simulink library "BLDC_controller_Lib_AccelerationBased"  (R2017b)
settings: Solver=VariableStepAuto  StartTime=0.0  StopTime=10.0  RelTol=1e-3
values from neighbouring files (symbols this model uses):
  a_elecAngle = 60    [init_model_Ffwd.m]
  a_elecPeriod = 360    [init_model_Ffwd.m]
  cf_speedCoef = round(f_ctrl * a_mechAngle * (pi/180) * (30/pi))    [init_model_Ffwd.m]
  cf_speedFilt = 0.20    (= 0.2)    [init_model_Ffwd.m]
  n_commAcvLo = 15    [init_model_Ffwd.m]
  n_commDeacvHi = 30    [init_model_Ffwd.m]
  r_sinPhaA_M1 = -sca_factor*sin(omega + pha_adv*(pi/180))    [init_model_Ffwd.m]
  r_sinPhaB_M1 = -sca_factor*sin(omega - 120*(pi/180) + pha_adv*(pi/180))    [init_model_Ffwd.m]
  r_sinPhaC_M1 = -sca_factor*sin(omega + 120*(pi/180) + pha_adv*(pi/180))    [init_model_Ffwd.m]
  r_trapPhaA_M1 = sca_factor*[ 1  1  1 -1 -1 -1  1]    [init_model_Ffwd.m]
  r_trapPhaB_M1 = sca_factor*[-1 -1  1  1  1 -1 -1]    [init_model_Ffwd.m]
  r_trapPhaC_M1 = sca_factor*[ 1 -1 -1 -1  1  1  1]    [init_model_Ffwd.m]
  vec_hallToPos = [0 2 0 1 4 3 5 0]    [init_model_Ffwd.m]
  z_commutMap_M1 = [-1 -1  0  1  1  0 ... (first row only)    [init_model_Ffwd.m]
  z_ctrlTypSel = 1    [init_model_Ffwd.m]
  z_maxCntRst = 2000    [init_model_Ffwd.m]
undefined symbols (not defined in the file or in its folder): a_phaAdv_M1, b_phaAdvEna, cf_speedSca, CTRL_COMM, r_commDCDeacv, r_sin3PhaA_M1, r_sin3PhaB_M1, r_sin3PhaC_M1, z_nrEdgeSpdAcv
libraries: BLDC_controller_Lib x3, simulink_extras x1
settings Model: Creator=37ef  LastModifiedBy=37ef

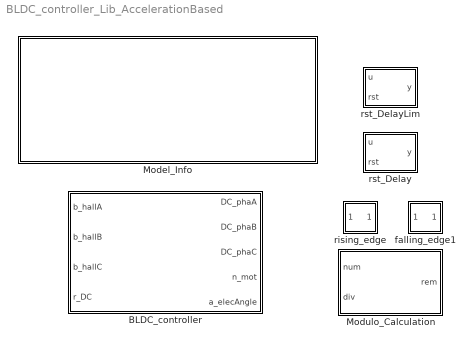
== system BLDC_controller_Lib_AccelerationBased ==
  BLDC_controller : Subsystem  SystemSampleTime=1e-5
  Model_Info : Subsystem
      mask DialogControl DescGroupVar Prompt: Model info
      mask DialogControl DescTextVar Prompt: This mask gives quick information about the model.
      mask Display:
      | info = Simulink.MDLInfo(bdroot);
      | file = dir([bdroot '.slx']);
      | % image('logo.png', [0.48, 0.55, 0.5, 0.4]);
      | text(0.05, 0.5, [...
      |         'MODEL INFO \n\n' ...
      |         'Version: ' info.ModelVersion '\n' ...
      |         'Author: ' 'Emanuel Feru' '\n' ...
      |         'Last modified by: ' info.LastModifiedBy '\n' ...
      |         'Last update: ' file.date '\n\n'], ...
      |         'horizontalAlignment', 'left', ...
      |         'verticalAlignment', 'middle');
      | 
      | color('blue');
      | text(0.95, 0.08, [...
      |         'Copyright © 2019 Emanuel FERU'], ...
      |         'horizontalAlignment', 'right', ...
      |         'verticalAlignment', 'bottom');
  Modulo_Calculation : Subsystem
  falling_edge1 : Subsystem  StopFcn=%tagged  TreatAsAtomicUnit=on  mask(Falling edge detection){}
      mask help:
      | Falling edge detection for a logic signal.
      | When a falling edge on the input signal is detected, the output switches to 1 during one time step.
      settings: RTWSystemCode=Nonreusable function
      mask Display: plot(0,0,100,100, [20 50 50 80], [90 90 10 10], [40 50 60], [55 45 55] )
  rising_edge : Subsystem  StopFcn=%tagged  TreatAsAtomicUnit=on  mask(Rising edge detection){}
      mask help:
      | Rising edge detection for a logic signal.
      | When a rising edge on the input signal is detected, the output switches to 1 during one time step.
      settings: RTWSystemCode=Nonreusable function
      mask Display: plot(0,0,100,100, [20 50 50 80], [10 10 90 90], [40 50 60], [45 55 45] )
  rst_Delay : Subsystem
      mask Display: dpoly(1,[1 0],'z')
  rst_DelayLim : Subsystem  mask{z_cntMaxLim=200}
      mask prompts: z_cntMaxLim "Maximum counter limit"
      mask Display: dpoly(1,[1 0],'z')

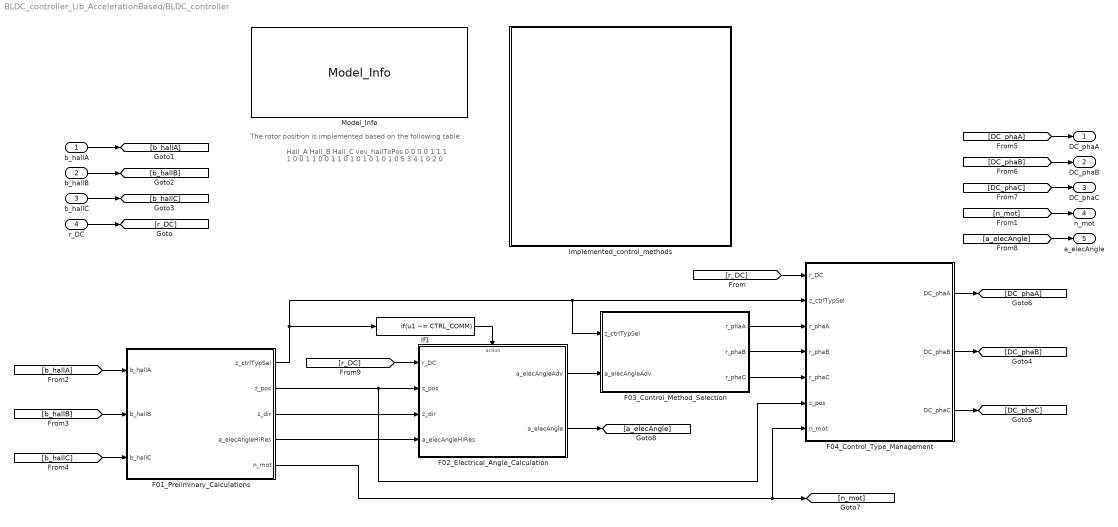
== system BLDC_controller_Lib_AccelerationBased/BLDC_controller ==
  note: The rotor position is implemented based on the following table:
  note: Hall_A
      | Hall_B
      | Hall_C
      | vev_hallToPos
      |
      | 0
      | 0
      | 0
      | 0
      | 1
      | 1
      | 1
      | 1
      | 0
      | 0
      | 1
      | 1
      | 0
      | 0
      | 1
      | 1
      | 0
      | 1
      | 0
      | 1
      | 0
      | 1
      | 0
      | 1
      | 0
      | 5
      | 3
      | 4
      | 1
      | 0
      | 2
      | 0
  "b_hallA " : Inport
  b_hallB : Inport  Port=2
  b_hallC : Inport  Port=3
  r_DC : Inport  Port=4
  F01_Preliminary_Calculations : Subsystem
  F02_Electrical_Angle_Calculation : Subsystem
  F03_Control_Method_Selection : Subsystem
  F04_Control_Type_Management : Subsystem
  If1 : If  IfExpression=u1 ~= CTRL_COMM  ShowElse=off
  Implemented_control_methods : Subsystem
      mask Display: image('control_methods.png')
  Model_Info : BLDC_controller_Lib/Model_Info
  DC_phaA : Outport
  DC_phaB : Outport  Port=2
  DC_phaC : Outport  Port=3
  n_mot : Outport  Port=4
  a_elecAngle : Outport  Port=5
  wires:
  "b_hallA "/1 -> [b_hallA]
  b_hallB/1 -> [b_hallB]
  b_hallC/1 -> [b_hallC]
  [n_mot] -> n_mot/1
  [DC_phaA] -> DC_phaA/1
  [b_hallA] -> F01_Preliminary_Calculations/1(b_hallA)
  [b_hallC] -> F01_Preliminary_Calculations/3(b_hallC)
  [b_hallB] -> F01_Preliminary_Calculations/2(b_hallB)
  F01_Preliminary_Calculations/2(z_pos) -> F04_Control_Type_Management/6(z_pos), F02_Electrical_Angle_Calculation/2(z_pos)
  F01_Preliminary_Calculations/3(z_dir) -> F02_Electrical_Angle_Calculation/3(z_dir)
  F01_Preliminary_Calculations/5("n_mot ") -> F04_Control_Type_Management/7(n_mot), [n_mot]
  F01_Preliminary_Calculations/4(a_elecAngleHiRes) -> F02_Electrical_Angle_Calculation/4(a_elecAngleHiRes)
  F01_Preliminary_Calculations/1(z_ctrlTypSel) -> F04_Control_Type_Management/2(z_ctrlTypSel), F03_Control_Method_Selection/1(z_ctrlTypSel), If1/1
  If1/1 -> F02_Electrical_Angle_Calculation/Action
  F02_Electrical_Angle_Calculation/1(a_elecAngleAdv) -> F03_Control_Method_Selection/2(a_elecAngleAdv)
  F03_Control_Method_Selection/1(r_phaA) -> F04_Control_Type_Management/3(r_phaA)
  F03_Control_Method_Selection/2(r_phaB) -> F04_Control_Type_Management/4(r_phaB)
  F03_Control_Method_Selection/3("r_phaC ") -> F04_Control_Type_Management/5(r_phaC)
  [r_DC] -> F04_Control_Type_Management/1(r_DC)
  F04_Control_Type_Management/1(DC_phaA) -> [DC_phaA]
  F04_Control_Type_Management/2(DC_phaB) -> [DC_phaB]
  F04_Control_Type_Management/3("DC_phaC ") -> [DC_phaC]
  [DC_phaB] -> DC_phaB/1
  [DC_phaC] -> DC_phaC/1
  r_DC/1 -> [r_DC]
  [a_elecAngle] -> a_elecAngle/1
  F02_Electrical_Angle_Calculation/2(a_elecAngle) -> [a_elecAngle]
  [r_DC] -> F02_Electrical_Angle_Calculation/1(r_DC)

== system BLDC_controller_Lib_AccelerationBased/Model_Info ==

== system BLDC_controller_Lib_AccelerationBased/Modulo_Calculation ==
  note: Modulo implementation: rem = num - div*(num/div)
      | Note : Division and multiplier has the setting 'Floor'
  num : Inport
  div : Inport  Port=2
  Divide2 : Product  Inputs=*/  OutDataTypeStr=Inherit: Same as first input
  Divide3 : Product  Inputs=**  OutDataTypeStr=Inherit: Same as first input
  Sum3 : Sum  Inputs=|+-  RndMeth=Simplest  OutDataTypeStr=Inherit: Same as first input
  rem : Outport
  wires:
  num/1 -> Sum3/1, Divide2/1
  Sum3/1 -> rem/1
  Divide3/1 -> Sum3/2
  div/1 -> Divide3/2, Divide2/2
  Divide2/1 -> Divide3/1

== system BLDC_controller_Lib_AccelerationBased/falling_edge1 ==
  Signal : Inport
  Logical Operator : Logic  Tag=struct('inputs','2','comment',struct('text','','placement',1),'logdata',struct('maxnumvals',inf,'plotchannels',[],'loggingmode',3,'channels',1),'operator','AND','output',struct('variable','','description','','name','$S_$B','address','','class','default','type','Bool','unit',''),'scalingvalid',0,'date',733067.68453166669)  OutDataTypeStr=boolean
  Logical Operator1 : Logic  Tag=struct('inputs','1','comment',struct('text','','placement',1),'logdata',struct('maxnumvals',inf,'plotchannels',[],'loggingmode',3,'channels',1),'operator','NOT','output',struct('variable','','description','','name','$S_$B','address','','class','default','type','Bool','unit',''),'scalingvalid',0,'date',733067.68453201384)  Operator=NOT  Inputs=1  OutDataTypeStr=boolean
  UnitDelay : UnitDelay  SampleTime=-1
      settings: AttributesFormatString=Te = %<SampleTime>\nIni=%<X0>
  Out : Outport
  wires:
  UnitDelay/1 -> Logical Operator/2
  Logical Operator1/1 -> Logical Operator/1
  Signal/1 -> UnitDelay/1, Logical Operator1/1
  Logical Operator/1 -> Out/1

== system BLDC_controller_Lib_AccelerationBased/rising_edge ==
  Signal : Inport
  Logical Operator : Logic  Tag=struct('inputs','2','comment',struct('text','','placement',1),'logdata',struct('maxnumvals',inf,'plotchannels',[],'loggingmode',3,'channels',1),'operator','AND','output',struct('variable','','description','','name','$S_$B','address','','class','default','type','Bool','unit',''),'scalingvalid',0,'date',733067.68458487268)  OutDataTypeStr=boolean
  Logical Operator1 : Logic  Tag=struct('inputs','1','comment',struct('text','','placement',1),'logdata',struct('maxnumvals',inf,'plotchannels',[],'loggingmode',3,'channels',1),'operator','NOT','output',struct('variable','','description','','name','$S_$B','address','','class','default','type','Bool','unit',''),'scalingvalid',0,'date',733067.68458533566)  Operator=NOT  Inputs=1  OutDataTypeStr=boolean
  UnitDelay : UnitDelay  SampleTime=-1
      settings: AttributesFormatString=Te = %<SampleTime>\nIni=%<X0>
  Out : Outport
  wires:
  UnitDelay/1 -> Logical Operator1/1
  Logical Operator1/1 -> Logical Operator/2
  Signal/1 -> Logical Operator/1, UnitDelay/1
  Logical Operator/1 -> Out/1

== system BLDC_controller_Lib_AccelerationBased/rst_Delay ==
  u : Inport
  rst : Inport  Port=2
  Constant23 : Constant  Value=0  OutDataTypeStr=Inherit: Inherit via back propagation
  Switch1 : Switch  Criteria=u2 ~= 0  OutDataTypeStr=Inherit: Inherit via back propagation  RndMeth=Simplest
  UnitDelay1 : UnitDelay  SampleTime=-1
  y : Outport
  wires:
  Switch1/1 -> y/1
  u/1 -> UnitDelay1/1
  UnitDelay1/1 -> Switch1/3
  rst/1 -> Switch1/2
  Constant23/1 -> Switch1/1

== system BLDC_controller_Lib_AccelerationBased/rst_DelayLim ==
  u : Inport
  rst : Inport  Port=2
  Constant1 : Constant  Value=z_cntMaxLim  OutDataTypeStr=Inherit: Inherit via back propagation
  Constant23 : Constant  Value=0  OutDataTypeStr=Inherit: Inherit via back propagation
  Relational Operator1 : RelationalOperator  Operator=<  OutDataTypeStr=boolean  RndMeth=Simplest
  Switch1 : Switch  Criteria=u2 ~= 0  OutDataTypeStr=Inherit: Inherit via back propagation  RndMeth=Simplest
  Switch2 : Switch  Criteria=u2 ~= 0  OutDataTypeStr=Inherit: Inherit via back propagation  RndMeth=Simplest
  UnitDelay1 : UnitDelay  InitialCondition=z_cntMaxLim  SampleTime=-1
  y : Outport
  wires:
  Switch1/1 -> y/1
  u/1 -> UnitDelay1/1
  rst/1 -> Switch1/2
  Constant23/1 -> Switch1/1
  UnitDelay1/1 -> Switch2/1, Relational Operator1/1
  Constant1/1 -> Switch2/3, Relational Operator1/2
  Relational Operator1/1 -> Switch2/2
  Switch2/1 -> Switch1/3

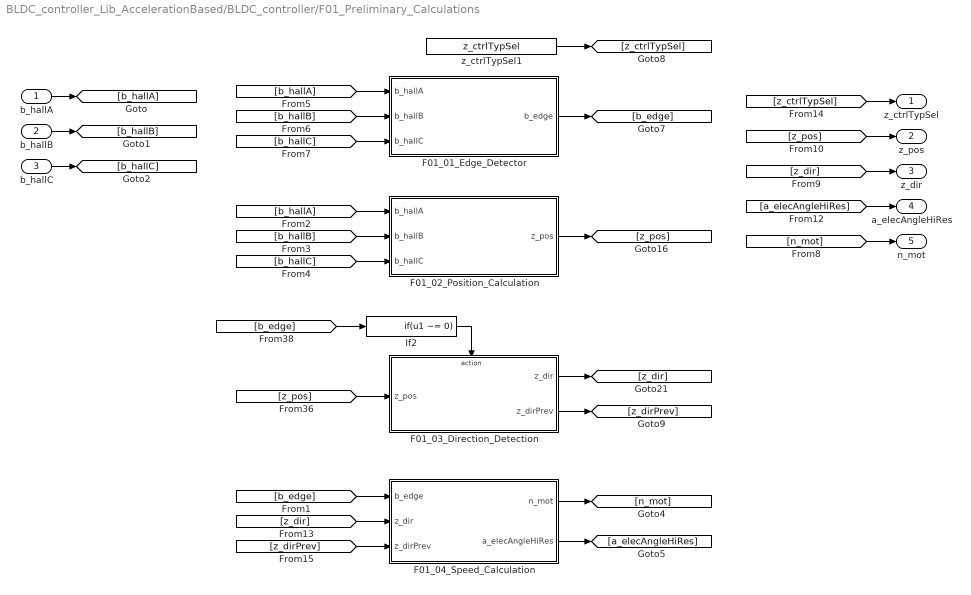
== system BLDC_controller_Lib_AccelerationBased/BLDC_controller/F01_Preliminary_Calculations ==
  b_hallA : Inport
  b_hallB : Inport  Port=2
  b_hallC : Inport  Port=3
  F01_01_Edge_Detector : Subsystem
  F01_02_Position_Calculation : Subsystem
  F01_03_Direction_Detection : Subsystem
  F01_04_Speed_Calculation : Subsystem
  If2 : If  IfExpression=u1 ~= 0  ShowElse=off
  z_ctrlTypSel1 : Constant  Value=z_ctrlTypSel  OutDataTypeStr=uint8
  z_ctrlTypSel : Outport  OutputWhenDisabled=reset  InitialOutput=0
  z_pos : Outport  Port=2  OutputWhenDisabled=reset  InitialOutput=0
  z_dir : Outport  Port=3  OutputWhenDisabled=reset  InitialOutput=0
  a_elecAngleHiRes : Outport  Port=4  OutputWhenDisabled=reset  InitialOutput=0
  "n_mot " : Outport  Port=5  OutputWhenDisabled=reset  InitialOutput=0
  wires:
  If2/1 -> F01_03_Direction_Detection/Action
  [b_edge] -> If2/1
  [z_pos] -> F01_03_Direction_Detection/1(z_pos)
  [b_hallA] -> F01_01_Edge_Detector/1(b_hallA)
  F01_01_Edge_Detector/1("b_edge ") -> [b_edge]
  F01_03_Direction_Detection/1(z_dir) -> [z_dir]
  [b_hallB] -> F01_01_Edge_Detector/2(b_hallB)
  [b_hallC] -> F01_01_Edge_Detector/3(b_hallC)
  b_hallA/1 -> [b_hallA]
  b_hallB/1 -> [b_hallB]
  b_hallC/1 -> [b_hallC]
  [b_hallC] -> F01_02_Position_Calculation/3(b_hallC)
  [b_hallB] -> F01_02_Position_Calculation/2(b_hallB)
  [b_hallA] -> F01_02_Position_Calculation/1(b_hallA)
  F01_02_Position_Calculation/1("z_pos ") -> [z_pos]
  [b_edge] -> F01_04_Speed_Calculation/1(b_edge)
  F01_04_Speed_Calculation/1(n_mot) -> [n_mot]
  [n_mot] -> "n_mot "/1
  [z_dir] -> z_dir/1
  [z_pos] -> z_pos/1
  F01_04_Speed_Calculation/2(a_elecAngleHiRes) -> [a_elecAngleHiRes]
  [a_elecAngleHiRes] -> a_elecAngleHiRes/1
  [z_dir] -> F01_04_Speed_Calculation/2(z_dir)
  [z_ctrlTypSel] -> z_ctrlTypSel/1
  z_ctrlTypSel1/1 -> [z_ctrlTypSel]
  F01_03_Direction_Detection/2(z_dirPrev) -> [z_dirPrev]
  [z_dirPrev] -> F01_04_Speed_Calculation/3(z_dirPrev)

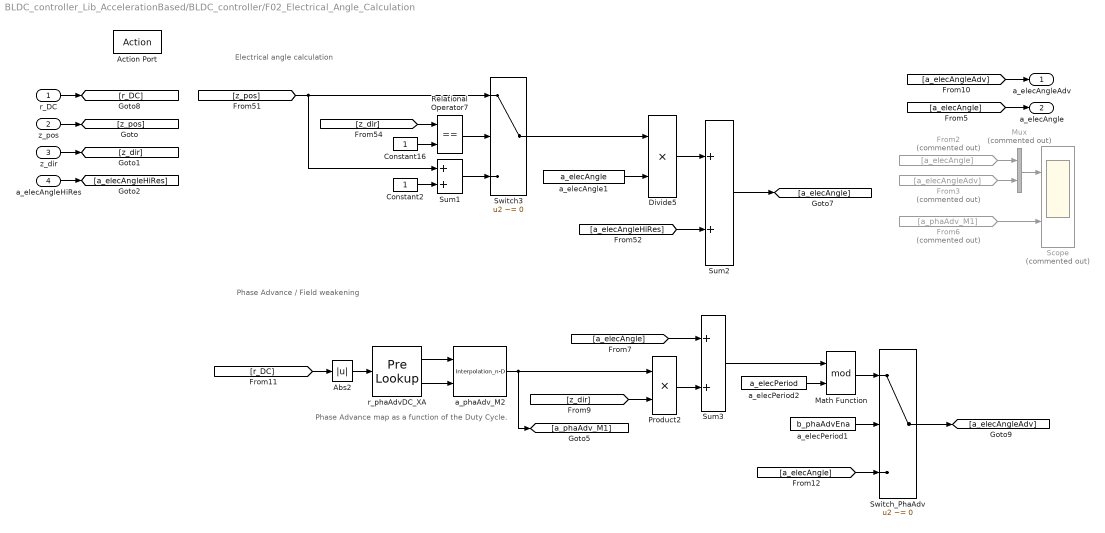
== system BLDC_controller_Lib_AccelerationBased/BLDC_controller/F02_Electrical_Angle_Calculation ==
  note: Electrical angle calculation
  note: Phase Advance / Field weakening
  note: Phase Advance map as a function of the Duty Cycle.
  r_DC : Inport
  z_pos : Inport  Port=2
  z_dir : Inport  Port=3
  a_elecAngleHiRes : Inport  Port=4
  Action Port : ActionPort
  Abs2 : Abs  ZeroCross=off  OutDataTypeStr=Inherit: Inherit via back propagation  RndMeth=Simplest
  Constant16 : Constant  OutDataTypeStr=Inherit: Inherit via back propagation
  Constant2 : Constant  OutDataTypeStr=Inherit: Inherit via back propagation
  Divide5 : Product  Inputs=**  OutDataTypeStr=int32  RndMeth=Simplest
  From2 : From  Commented=on  GotoTag=a_elecAngle
  From3 : From  Commented=on  GotoTag=a_elecAngleAdv
  From6 : From  Commented=on  GotoTag=a_phaAdv_M1
  Math Function : Math  Operator=mod  SaturateOnIntegerOverflow=on
  Mux : Mux  Commented=on  Inputs=2
  Product2 : Product  RndMeth=Simplest  OutDataTypeStr=Inherit: Same as first input
  Relational Operator7 : RelationalOperator  Operator===  OutDataTypeStr=boolean  RndMeth=Simplest
  Scope : Scope  Commented=on  NumInputPorts=2
  Sum1 : Sum  RndMeth=Simplest  OutDataTypeStr=Inherit: Same as first input
  Sum2 : Sum  RndMeth=Simplest  OutDataTypeStr=Inherit: Same as first input
  Sum3 : Sum  RndMeth=Simplest  OutDataTypeStr=Inherit: Same as first input
  Switch3 : Switch  Criteria=u2 ~= 0  OutDataTypeStr=Inherit: Inherit via back propagation  RndMeth=Zero
  Switch_PhaAdv : Switch  Criteria=u2 ~= 0  OutDataTypeStr=Inherit: Inherit via back propagation  RndMeth=Zero
  a_elecAngle1 : Constant  Value=a_elecAngle  OutDataTypeStr=int32
  a_elecPeriod1 : Constant  Value=b_phaAdvEna  OutDataTypeStr=boolean
  a_elecPeriod2 : Constant  Value=a_elecPeriod  OutDataTypeStr=Inherit: Inherit via back propagation
  a_phaAdv_M2 : Interpolation_n-D  NumberOfTableDimensions=1  Table=a_phaAdv_M1  ExtrapMethod=Clip  OutDataTypeStr=int16  InternalRulePriority=Speed  RndMeth=Simplest
      settings: InputPortMap=u0,u1
  r_phaAdvDC_XA : PreLookup  BreakpointsData=r_phaAdvDC_XA  IndexSearchMethod=Evenly spaced points  BeginIndexSearchUsingPreviousIndexResult=on  IndexDataTypeStr=uint8  RndMeth=Simplest
  a_elecAngleAdv : Outport  OutputWhenDisabled=reset  InitialOutput=0
  a_elecAngle : Outport  Port=2  OutputWhenDisabled=reset  InitialOutput=0
  wires:
  a_phaAdv_M2/1 -> [a_phaAdv_M1], Product2/1
  [z_dir] -> Product2/2
  [a_elecAngleHiRes] -> Sum2/2
  z_pos/1 -> [z_pos]
  z_dir/1 -> [z_dir]
  a_elecAngleHiRes/1 -> [a_elecAngleHiRes]
  Switch3/1 -> Divide5/1
  [z_pos] -> Sum1/1, Switch3/1
  Relational Operator7/1 -> Switch3/2
  [z_dir] -> Relational Operator7/1
  Divide5/1 -> Sum2/1
  Constant16/1 -> Relational Operator7/2
  a_elecAngle1/1 -> Divide5/2
  Constant2/1 -> Sum1/2
  Sum2/1 -> [a_elecAngle]
  Mux/1 -> Scope/1
  From2/1 -> Mux/1
  From3/1 -> Mux/2
  Sum1/1 -> Switch3/3
  [a_elecAngle] -> a_elecAngle/1
  [a_elecAngleAdv] -> a_elecAngleAdv/1
  From6/1 -> Scope/2
  a_elecPeriod1/1 -> Switch_PhaAdv/2
  r_phaAdvDC_XA/2 -> a_phaAdv_M2/2
  r_phaAdvDC_XA/1 -> a_phaAdv_M2/1
  [a_elecAngle] -> Switch_PhaAdv/3
  r_DC/1 -> [r_DC]
  Switch_PhaAdv/1 -> [a_elecAngleAdv]
  Product2/1 -> Sum3/2
  [a_elecAngle] -> Sum3/1
  [r_DC] -> Abs2/1
  Abs2/1 -> r_phaAdvDC_XA/1
  a_elecPeriod2/1 -> Math Function/2
  Math Function/1 -> Switch_PhaAdv/1
  Sum3/1 -> Math Function/1

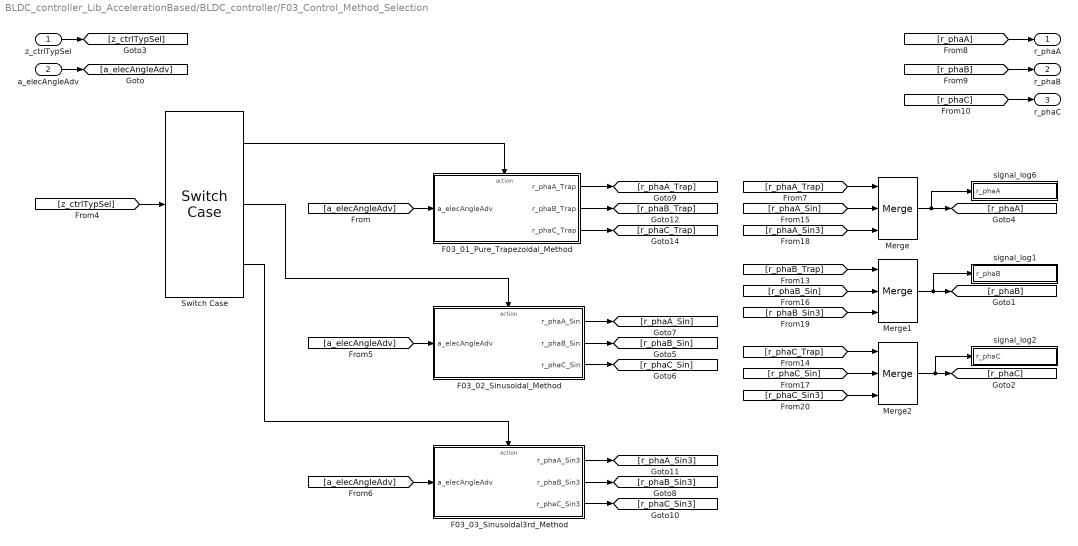
== system BLDC_controller_Lib_AccelerationBased/BLDC_controller/F03_Control_Method_Selection ==
  z_ctrlTypSel : Inport
  a_elecAngleAdv : Inport  Port=2
  F03_01_Pure_Trapezoidal_Method : Subsystem
  F03_02_Sinusoidal_Method : Subsystem
  F03_03_Sinusoidal3rd_Method : Subsystem
  Merge : Merge  Inputs=3
  Merge1 : Merge  Inputs=3
  Merge2 : Merge  Inputs=3
  Switch Case : SwitchCase  CaseConditions={CTRL_TRAP, CTRL_SIN, CTRL_SIN3}  ShowDefaultCase=off
  signal_log1 : Subsystem
  signal_log2 : Subsystem
  signal_log6 : Subsystem
  r_phaA : Outport  OutputWhenDisabled=reset  InitialOutput=0
  r_phaB : Outport  Port=2  OutputWhenDisabled=reset  InitialOutput=0
  "r_phaC " : Outport  Port=3  OutputWhenDisabled=reset  InitialOutput=0
  wires:
  [r_phaA] -> r_phaA/1
  [r_phaB] -> r_phaB/1
  [r_phaC] -> "r_phaC "/1
  a_elecAngleAdv/1 -> [a_elecAngleAdv]
  F03_01_Pure_Trapezoidal_Method/1(r_phaA_Trap) -> [r_phaA_Trap]
  [z_ctrlTypSel] -> Switch Case/1
  [a_elecAngleAdv] -> F03_01_Pure_Trapezoidal_Method/1(a_elecAngleAdv)
  Switch Case/1 -> F03_01_Pure_Trapezoidal_Method/Action
  [a_elecAngleAdv] -> F03_02_Sinusoidal_Method/1(a_elecAngleAdv)
  [a_elecAngleAdv] -> F03_03_Sinusoidal3rd_Method/1(a_elecAngleAdv)
  Switch Case/2 -> F03_02_Sinusoidal_Method/Action
  Switch Case/3 -> F03_03_Sinusoidal3rd_Method/Action
  F03_01_Pure_Trapezoidal_Method/2(r_phaB_Trap) -> [r_phaB_Trap]
  F03_01_Pure_Trapezoidal_Method/3(r_phaC_Trap) -> [r_phaC_Trap]
  F03_02_Sinusoidal_Method/3(r_phaC_Sin) -> [r_phaC_Sin]
  F03_02_Sinusoidal_Method/2(r_phaB_Sin) -> [r_phaB_Sin]
  F03_02_Sinusoidal_Method/1(r_phaA_Sin) -> [r_phaA_Sin]
  F03_03_Sinusoidal3rd_Method/3(r_phaC_Sin3) -> [r_phaC_Sin3]
  F03_03_Sinusoidal3rd_Method/2(r_phaB_Sin3) -> [r_phaB_Sin3]
  F03_03_Sinusoidal3rd_Method/1(r_phaA_Sin3) -> [r_phaA_Sin3]
  Merge/1 -> signal_log6/1(r_phaA), [r_phaA]
  Merge1/1 -> signal_log1/1(r_phaB), [r_phaB]
  Merge2/1 -> signal_log2/1(r_phaC), [r_phaC]
  [r_phaA_Trap] -> Merge/1
  z_ctrlTypSel/1 -> [z_ctrlTypSel]
  [r_phaA_Sin] -> Merge/2
  [r_phaA_Sin3] -> Merge/3
  [r_phaB_Trap] -> Merge1/1
  [r_phaB_Sin] -> Merge1/2
  [r_phaC_Trap] -> Merge2/1
  [r_phaB_Sin3] -> Merge1/3
  [r_phaC_Sin] -> Merge2/2
  [r_phaC_Sin3] -> Merge2/3

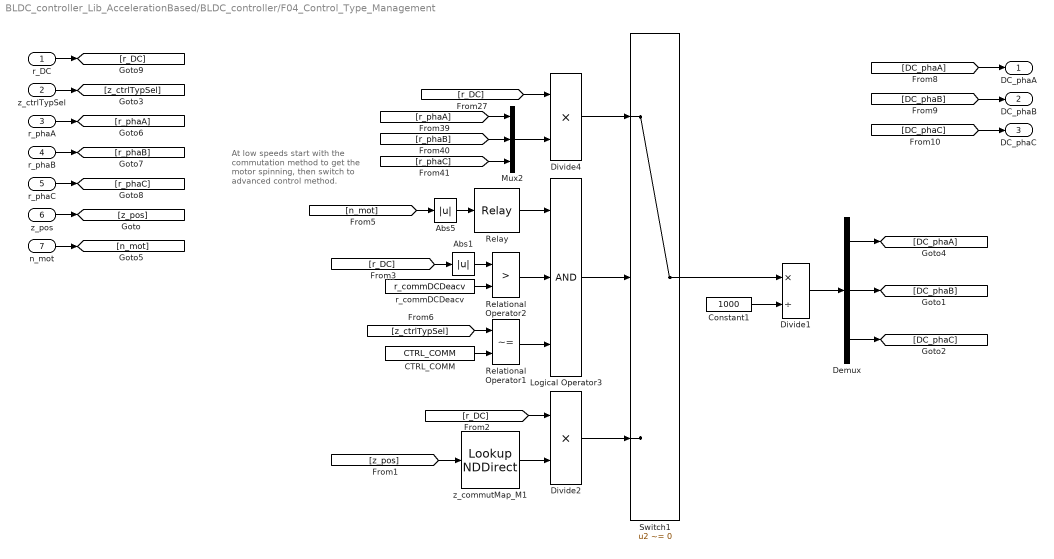
== system BLDC_controller_Lib_AccelerationBased/BLDC_controller/F04_Control_Type_Management ==
  note: At low speeds start with the commutation method to get the motor spinning, then switch to advanced control method.
  r_DC : Inport
  z_ctrlTypSel : Inport  Port=2
  r_phaA : Inport  Port=3
  r_phaB : Inport  Port=4
  r_phaC : Inport  Port=5
  z_pos : Inport  Port=6
  n_mot : Inport  Port=7
  Abs1 : Abs  OutDataTypeStr=Inherit: Inherit via back propagation  RndMeth=Zero
  Abs5 : Abs  OutDataTypeStr=Inherit: Inherit via back propagation  RndMeth=Zero
  CTRL_COMM : Constant  Value=CTRL_COMM  OutDataTypeStr=Inherit: Inherit via back propagation
  Constant1 : Constant  Value=1000  OutDataTypeStr=Inherit: Inherit via back propagation
  Demux : Demux  Outputs=3
  Divide1 : Product  Inputs=*/  RndMeth=Simplest  OutDataTypeStr=Inherit: Same as first input
  Divide2 : Product  Inputs=**  RndMeth=Simplest  OutDataTypeStr=Inherit: Same as first input
  Divide4 : Product  Inputs=**  RndMeth=Simplest  OutDataTypeStr=Inherit: Same as first input
  Logical Operator3 : Logic  Inputs=3  AllPortsSameDT=off  OutDataTypeStr=boolean
  Mux2 : Mux  Inputs=3
  Relational Operator1 : RelationalOperator  Operator=~=  OutDataTypeStr=boolean  RndMeth=Simplest
  Relational Operator2 : RelationalOperator  Operator=>  OutDataTypeStr=boolean  RndMeth=Simplest
  Relay : Relay  OnSwitchValue=n_commDeacvHi  OffSwitchValue=n_commAcvLo  OutDataTypeStr=boolean
  Switch1 : Switch  Criteria=u2 ~= 0  OutDataTypeStr=Inherit: Inherit via back propagation  RndMeth=Zero
  r_commDCDeacv : Constant  Value=r_commDCDeacv  OutDataTypeStr=Inherit: Inherit via back propagation
  z_commutMap_M1 : LookupNDDirect  InputsSelectThisObjectFromTable=Column  Table=z_commutMap_M1  DiagnosticForOutOfRangeInput=None  TableDataTypeStr=int16
  DC_phaA : Outport  OutputWhenDisabled=reset  InitialOutput=0
  DC_phaB : Outport  Port=2  OutputWhenDisabled=reset  InitialOutput=0
  "DC_phaC " : Outport  Port=3  OutputWhenDisabled=reset  InitialOutput=0
  wires:
  z_ctrlTypSel/1 -> [z_ctrlTypSel]
  Demux/3 -> [DC_phaC]
  Demux/2 -> [DC_phaB]
  Demux/1 -> [DC_phaA]
  z_pos/1 -> [z_pos]
  [DC_phaC] -> "DC_phaC "/1
  [DC_phaB] -> DC_phaB/1
  [DC_phaA] -> DC_phaA/1
  Switch1/1 -> Divide1/1
  Relay/1 -> Logical Operator3/1
  [z_ctrlTypSel] -> Relational Operator1/1
  CTRL_COMM/1 -> Relational Operator1/2
  Abs5/1 -> Relay/1
  [z_pos] -> z_commutMap_M1/1
  Divide1/1 -> Demux/1
  n_mot/1 -> [n_mot]
  r_phaA/1 -> [r_phaA]
  r_phaB/1 -> [r_phaB]
  r_phaC/1 -> [r_phaC]
  r_DC/1 -> [r_DC]
  [r_phaA] -> Mux2/1
  [r_phaB] -> Mux2/2
  [r_phaC] -> Mux2/3
  Mux2/1 -> Divide4/2
  Divide4/1 -> Switch1/1
  Constant1/1 -> Divide1/2
  [r_DC] -> Divide2/1
  z_commutMap_M1/1 -> Divide2/2
  Divide2/1 -> Switch1/3
  [n_mot] -> Abs5/1
  Logical Operator3/1 -> Switch1/2
  [r_DC] -> Divide4/1
  [r_DC] -> Abs1/1
  r_commDCDeacv/1 -> Relational Operator2/2
  Relational Operator1/1 -> Logical Operator3/3
  Relational Operator2/1 -> Logical Operator3/2
  Abs1/1 -> Relational Operator2/1

== system BLDC_controller_Lib_AccelerationBased/BLDC_controller/Implemented_control_methods ==

== system BLDC_controller_Lib_AccelerationBased/BLDC_controller/F01_Preliminary_Calculations/F01_01_Edge_Detector ==
  b_hallA : Inport
  b_hallB : Inport  Port=2
  b_hallC : Inport  Port=3
  Logical Operator : Logic  Operator=XOR  Inputs=6  AllPortsSameDT=off  OutDataTypeStr=boolean
  UnitDelay : UnitDelay  SampleTime=-1
  UnitDelay1 : UnitDelay  SampleTime=-1
  UnitDelay2 : UnitDelay  SampleTime=-1
  "b_edge " : Outport  OutputWhenDisabled=reset  InitialOutput=0
  wires:
  b_hallA/1 -> UnitDelay/1, Logical Operator/1
  b_hallC/1 -> UnitDelay2/1, Logical Operator/3
  b_hallB/1 -> UnitDelay1/1, Logical Operator/2
  Logical Operator/1 -> "b_edge "/1
  UnitDelay1/1 -> Logical Operator/5
  UnitDelay2/1 -> Logical Operator/6
  UnitDelay/1 -> Logical Operator/4

== system BLDC_controller_Lib_AccelerationBased/BLDC_controller/F01_Preliminary_Calculations/F01_02_Position_Calculation ==
  note: This calculates the low resolution position based on Hall sensors.
  b_hallA : Inport
  b_hallB : Inport  Port=2
  b_hallC : Inport  Port=3
  Selector : Selector  IndexMode=Zero-based  InputPortWidth=length(vec_hallToPos)  IndexOptions=Index vector (port)  Indices=[1 3]  OutputSizes=1
  Sum : Sum  Inputs=+++  RndMeth=Simplest  OutDataTypeStr=Inherit: Same as first input
  g_Ha : Gain  Gain=4  OutDataTypeStr=Inherit: Inherit via back propagation  RndMeth=Zero  ParamDataTypeStr=Inherit: Same as input
  g_Hb : Gain  Gain=2  OutDataTypeStr=Inherit: Inherit via back propagation  RndMeth=Simplest  ParamDataTypeStr=Inherit: Same as input
  vec_hallToPos : Constant  Value=vec_hallToPos  OutDataTypeStr=int8
  "z_pos " : Outport  OutputWhenDisabled=reset  InitialOutput=0
  wires:
  b_hallC/1 -> Sum/3
  g_Ha/1 -> Sum/1
  g_Hb/1 -> Sum/2
  Sum/1 -> Selector/2
  b_hallA/1 -> g_Ha/1
  b_hallB/1 -> g_Hb/1
  vec_hallToPos/1 -> Selector/1
  Selector/1 -> "z_pos "/1

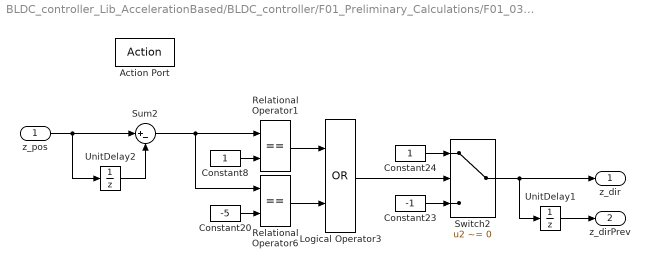
== system BLDC_controller_Lib_AccelerationBased/BLDC_controller/F01_Preliminary_Calculations/F01_03_Direction_Detection ==
  z_pos : Inport
  Action Port : ActionPort
  Constant20 : Constant  Value=-5  OutDataTypeStr=Inherit: Inherit via back propagation
  Constant23 : Constant  Value=-1  OutDataTypeStr=int8
  Constant24 : Constant  OutDataTypeStr=int8
  Constant8 : Constant  OutDataTypeStr=Inherit: Inherit via back propagation
  Logical Operator3 : Logic  Operator=OR  AllPortsSameDT=off  OutDataTypeStr=boolean
  Relational Operator1 : RelationalOperator  Operator===  OutDataTypeStr=boolean  RndMeth=Simplest
  Relational Operator6 : RelationalOperator  Operator===  OutDataTypeStr=boolean  RndMeth=Simplest
  Sum2 : Sum  Inputs=|+-  RndMeth=Zero  InputSameDT=on  OutDataTypeStr=Inherit: Same as first input
  Switch2 : Switch  Criteria=u2 ~= 0  OutDataTypeStr=Inherit: Inherit via back propagation  RndMeth=Simplest
  UnitDelay1 : UnitDelay  SampleTime=-1
  UnitDelay2 : UnitDelay  SampleTime=-1
  z_dir : Outport
  z_dirPrev : Outport  Port=2
  wires:
  UnitDelay2/1 -> Sum2/2
  Relational Operator1/1 -> Logical Operator3/1
  Constant8/1 -> Relational Operator1/2
  Sum2/1 -> Relational Operator6/1, Relational Operator1/1
  Relational Operator6/1 -> Logical Operator3/2
  Constant20/1 -> Relational Operator6/2
  Constant24/1 -> Switch2/1
  Constant23/1 -> Switch2/3
  Logical Operator3/1 -> Switch2/2
  Switch2/1 -> z_dir/1, UnitDelay1/1
  z_pos/1 -> Sum2/1, UnitDelay2/1
  UnitDelay1/1 -> z_dirPrev/1

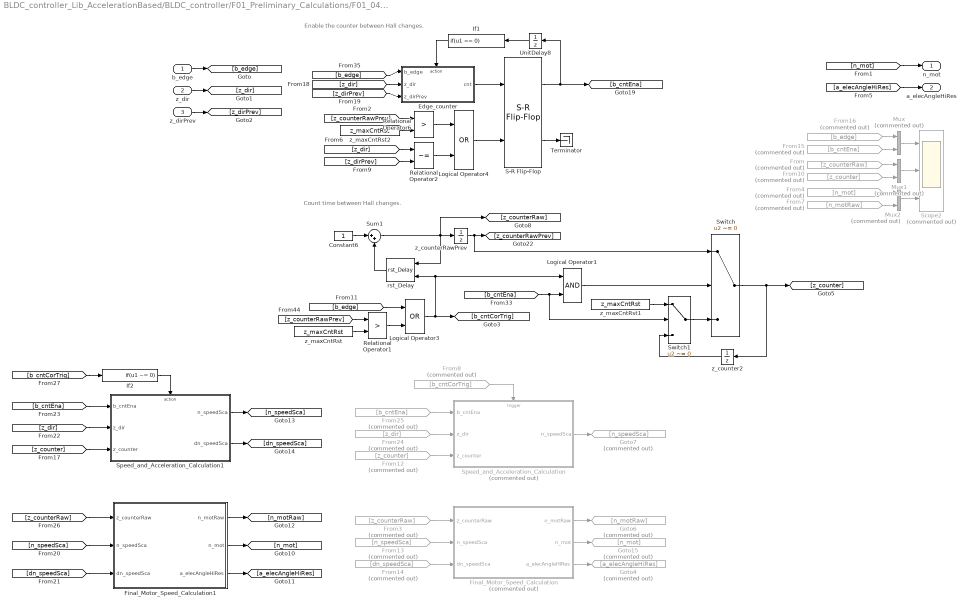
== system BLDC_controller_Lib_AccelerationBased/BLDC_controller/F01_Preliminary_Calculations/F01_04_Speed_Calculation ==
  note: Count time between Hall changes.
  note: Enable the counter between Hall changes.
  b_edge : Inport
  z_dir : Inport  Port=2
  z_dirPrev : Inport  Port=3
  Constant6 : Constant  OutDataTypeStr=Inherit: Inherit via back propagation
  Edge_counter : Subsystem
  Final_Motor_Speed_Calculation : Subsystem  Commented=on
  Final_Motor_Speed_Calculation1 : Subsystem
  From : From  Commented=on  GotoTag=z_counterRaw
  From10 : From  Commented=on  GotoTag=z_counter
  From12 : From  Commented=on  GotoTag=z_counter
  From13 : From  Commented=on  GotoTag=n_speedSca
  From14 : From  Commented=on  GotoTag=dn_speedSca
  From15 : From  Commented=on  GotoTag=b_cntEna
  From16 : From  Commented=on  GotoTag=b_edge
  From24 : From  Commented=on  GotoTag=z_dir
  From25 : From  Commented=on  GotoTag=b_cntEna
  From3 : From  Commented=on  GotoTag=z_counterRaw
  From4 : From  Commented=on  GotoTag=n_mot
  From7 : From  Commented=on  GotoTag=n_motRaw
  From8 : From  Commented=on  GotoTag=b_cntCorTrig
  Goto15 : Goto  Commented=on  GotoTag=n_mot
  Goto4 : Goto  Commented=on  GotoTag=a_elecAngleHiRes
  Goto6 : Goto  Commented=on  GotoTag=n_motRaw
  Goto7 : Goto  Commented=on  GotoTag=n_speedSca
  If1 : If  IfExpression=u1 == 0  ShowElse=off
  If2 : If  IfExpression=u1 ~= 0  ShowElse=off
  Logical Operator1 : Logic  AllPortsSameDT=off  OutDataTypeStr=boolean
  Logical Operator3 : Logic  Operator=OR  AllPortsSameDT=off  OutDataTypeStr=boolean
  Logical Operator4 : Logic  Operator=OR  AllPortsSameDT=off  OutDataTypeStr=boolean
  Mux : Mux  Commented=on  Inputs=2
  Mux1 : Mux  Commented=on  Inputs=2
  Mux2 : Mux  Commented=on  Inputs=2
  Relational Operator1 : RelationalOperator  Operator=>  OutDataTypeStr=boolean  RndMeth=Simplest
  Relational Operator2 : RelationalOperator  Operator=~=  OutDataTypeStr=boolean  RndMeth=Simplest
  Relational Operator6 : RelationalOperator  Operator=>  OutDataTypeStr=boolean  RndMeth=Simplest
  S-R Flip-Flop : simulink_extras/Flip Flops/S-R Flip-Flop  initial_condition=0
  Scope2 : Scope  Commented=on  NumInputPorts=3
  Speed_and_Acceleration_Calculation : Subsystem  Commented=on
  Speed_and_Acceleration_Calculation1 : Subsystem
  Sum1 : Sum  Inputs=|++  RndMeth=Simplest  InputSameDT=on  OutDataTypeStr=Inherit: Same as first input
  Switch : Switch  Criteria=u2 ~= 0  OutDataTypeStr=Inherit: Inherit via back propagation  RndMeth=Simplest
  Switch1 : Switch  Criteria=u2 ~= 0  OutDataTypeStr=Inherit: Inherit via back propagation  RndMeth=Simplest
  Terminator : Terminator
      settings: Tag=Controls_Lib  Description=Terminator  CopyFcn=Lib_CopyFcn(gcb);  PreDeleteFcn=Lib_PreDeleteFcn(gcb);
  UnitDelay8 : UnitDelay  SampleTime=-1
  rst_Delay : BLDC_controller_Lib/rst_Delay
  z_counter2 : UnitDelay  InitialCondition=z_maxCntRst  SampleTime=-1
  z_counterRawPrev : UnitDelay  SampleTime=-1
  z_maxCntRst : Constant  Value=z_maxCntRst  OutDataTypeStr=int32
  z_maxCntRst1 : Constant  Value=z_maxCntRst  OutDataTypeStr=int32
  z_maxCntRst2 : Constant  Value=z_maxCntRst  OutDataTypeStr=int32
  n_mot : Outport
  a_elecAngleHiRes : Outport  Port=2
  wires:
  If2/1 -> Speed_and_Acceleration_Calculation1/Action
  [b_cntCorTrig] -> If2/1
  If1/1 -> Edge_counter/Action
  Relational Operator2/1 -> Logical Operator4/2
  [b_cntEna] -> Logical Operator1/2, Switch1/2
  From8/1 -> Speed_and_Acceleration_Calculation/Trigger
  From12/1 -> Speed_and_Acceleration_Calculation/3(z_counter)
  Final_Motor_Speed_Calculation1/2(n_mot) -> [n_mot]
  Final_Motor_Speed_Calculation1/1(n_motRaw) -> [n_motRaw]
  [z_counter] -> Speed_and_Acceleration_Calculation1/3(z_counter)
  [z_dir] -> Speed_and_Acceleration_Calculation1/2(z_dir)
  [b_cntEna] -> Speed_and_Acceleration_Calculation1/1(b_cntEna)
  [z_counterRaw] -> Final_Motor_Speed_Calculation1/1(z_counterRaw)
  Final_Motor_Speed_Calculation1/3(a_elecAngleHiRes) -> [a_elecAngleHiRes]
  Speed_and_Acceleration_Calculation1/1(n_speedSca) -> [n_speedSca]
  Speed_and_Acceleration_Calculation1/2(dn_speedSca) -> [dn_speedSca]
  [n_speedSca] -> Final_Motor_Speed_Calculation1/2(n_speedSca)
  [dn_speedSca] -> Final_Motor_Speed_Calculation1/3(dn_speedSca)
  [z_dirPrev] -> Relational Operator2/2
  [z_dir] -> Relational Operator2/1
  Relational Operator6/1 -> Logical Operator4/1
  From14/1 -> Final_Motor_Speed_Calculation/3(dn_speedSca)
  From13/1 -> Final_Motor_Speed_Calculation/2(n_speedSca)
  Speed_and_Acceleration_Calculation/1(n_speedSca) -> Goto7/1
  Final_Motor_Speed_Calculation/3(a_elecAngleHiRes) -> Goto4/1
  From3/1 -> Final_Motor_Speed_Calculation/1(z_counterRaw)
  From25/1 -> Speed_and_Acceleration_Calculation/1(b_cntEna)
  From24/1 -> Speed_and_Acceleration_Calculation/2(z_dir)
  From7/1 -> Mux2/2
  Final_Motor_Speed_Calculation/1(n_motRaw) -> Goto6/1
  Logical Operator1/1 -> Switch/2
  Mux2/1 -> Scope2/3
  From4/1 -> Mux2/1
  Final_Motor_Speed_Calculation/2(n_mot) -> Goto15/1
  z_maxCntRst2/1 -> Relational Operator6/2
  [z_counterRawPrev] -> Relational Operator6/1
  [b_edge] -> Logical Operator3/1
  Switch1/1 -> Switch/3
  z_maxCntRst1/1 -> Switch1/1
  Mux1/1 -> Scope2/2
  From/1 -> Mux1/1
  From10/1 -> Mux1/2
  From15/1 -> Mux/2
  From16/1 -> Mux/1
  Mux/1 -> Scope2/1
  Relational Operator1/1 -> Logical Operator3/2
  [z_counterRawPrev] -> Relational Operator1/1
  z_counter2/1 -> Switch1/3
  z_counterRawPrev/1 -> [z_counterRawPrev], Switch/1
  Logical Operator3/1 -> Logical Operator1/1, rst_Delay/2, [b_cntCorTrig]
  z_maxCntRst/1 -> Relational Operator1/2
  Constant6/1 -> Sum1/1
  Sum1/1 -> rst_Delay/1, z_counterRawPrev/1, [z_counterRaw]
  b_edge/1 -> [b_edge]
  [n_mot] -> n_mot/1
  [a_elecAngleHiRes] -> a_elecAngleHiRes/1
  z_dir/1 -> [z_dir]
  z_dirPrev/1 -> [z_dirPrev]
  rst_Delay/1 -> Sum1/2
  S-R Flip-Flop/2 -> Terminator/1
  [z_dirPrev] -> Edge_counter/3(z_dirPrev)
  [z_dir] -> Edge_counter/2(z_dir)
  Edge_counter/1(cnt) -> S-R Flip-Flop/1
  S-R Flip-Flop/1 -> [b_cntEna], UnitDelay8/1
  UnitDelay8/1 -> If1/1
  Logical Operator4/1 -> S-R Flip-Flop/2
  [b_edge] -> Edge_counter/1(b_edge)
  Switch/1 -> [z_counter], z_counter2/1

== system BLDC_controller_Lib_AccelerationBased/BLDC_controller/F03_Control_Method_Selection/F03_01_Pure_Trapezoidal_Method ==
  a_elecAngleAdv : Inport
  Action Port : ActionPort  InitializeStates=reset
  a_trapElecAngle_XA : PreLookup  BreakpointsData=a_trapElecAngle_XA  IndexSearchMethod=Evenly spaced points  BeginIndexSearchUsingPreviousIndexResult=on  IndexDataTypeStr=uint8  RndMeth=Simplest
  r_trapPhaA_M1 : Interpolation_n-D  NumberOfTableDimensions=1  Table=r_trapPhaA_M1  ExtrapMethod=Clip  RemoveProtectionIndex=on  OutDataTypeStr=int16  InternalRulePriority=Speed  RndMeth=Simplest
      settings: InputPortMap=u0,u1
  r_trapPhaB_M1 : Interpolation_n-D  NumberOfTableDimensions=1  Table=r_trapPhaB_M1  ExtrapMethod=Clip  RemoveProtectionIndex=on  OutDataTypeStr=int16  InternalRulePriority=Speed  RndMeth=Simplest
      settings: InputPortMap=u0,u1
  r_trapPhaC_M1 : Interpolation_n-D  NumberOfTableDimensions=1  Table=r_trapPhaC_M1  ExtrapMethod=Clip  RemoveProtectionIndex=on  OutDataTypeStr=int16  InternalRulePriority=Speed  RndMeth=Simplest
      settings: InputPortMap=u0,u1
  r_phaA_Trap : Outport
  r_phaB_Trap : Outport  Port=2
  r_phaC_Trap : Outport  Port=3
  wires:
  a_trapElecAngle_XA/1 -> r_trapPhaA_M1/1, r_trapPhaC_M1/1, r_trapPhaB_M1/1
  a_trapElecAngle_XA/2 -> r_trapPhaC_M1/2, r_trapPhaB_M1/2, r_trapPhaA_M1/2
  r_trapPhaA_M1/1 -> r_phaA_Trap/1
  r_trapPhaB_M1/1 -> r_phaB_Trap/1
  r_trapPhaC_M1/1 -> r_phaC_Trap/1
  a_elecAngleAdv/1 -> a_trapElecAngle_XA/1

== system BLDC_controller_Lib_AccelerationBased/BLDC_controller/F03_Control_Method_Selection/F03_02_Sinusoidal_Method ==
  a_elecAngleAdv : Inport
  Action Port : ActionPort  InitializeStates=reset
  a_sinElecAngle_XA : PreLookup  BreakpointsData=a_sinElecAngle_XA  IndexSearchMethod=Evenly spaced points  BeginIndexSearchUsingPreviousIndexResult=on  IndexDataTypeStr=uint8  RndMeth=Simplest
  r_sinPhaA_M1 : Interpolation_n-D  NumberOfTableDimensions=1  Table=r_sinPhaA_M1  ExtrapMethod=Clip  RemoveProtectionIndex=on  OutDataTypeStr=int16  InternalRulePriority=Speed  RndMeth=Simplest
      settings: InputPortMap=u0,u1
  r_sinPhaB_M1 : Interpolation_n-D  NumberOfTableDimensions=1  Table=r_sinPhaB_M1  ExtrapMethod=Clip  RemoveProtectionIndex=on  OutDataTypeStr=int16  InternalRulePriority=Speed  RndMeth=Simplest
      settings: InputPortMap=u0,u1
  r_sinPhaC_M1 : Interpolation_n-D  NumberOfTableDimensions=1  Table=r_sinPhaC_M1  ExtrapMethod=Clip  RemoveProtectionIndex=on  OutDataTypeStr=int16  InternalRulePriority=Speed  RndMeth=Simplest
      settings: InputPortMap=u0,u1
  r_phaA_Sin : Outport
  r_phaB_Sin : Outport  Port=2
  r_phaC_Sin : Outport  Port=3
  wires:
  a_sinElecAngle_XA/2 -> r_sinPhaA_M1/2, r_sinPhaB_M1/2, r_sinPhaC_M1/2
  a_elecAngleAdv/1 -> a_sinElecAngle_XA/1
  r_sinPhaC_M1/1 -> r_phaC_Sin/1
  r_sinPhaB_M1/1 -> r_phaB_Sin/1
  r_sinPhaA_M1/1 -> r_phaA_Sin/1
  a_sinElecAngle_XA/1 -> r_sinPhaA_M1/1, r_sinPhaB_M1/1, r_sinPhaC_M1/1

== system BLDC_controller_Lib_AccelerationBased/BLDC_controller/F03_Control_Method_Selection/F03_03_Sinusoidal3rd_Method ==
  a_elecAngleAdv : Inport
  Action Port : ActionPort  InitializeStates=reset
  a_sinElecAngle_XA : PreLookup  BreakpointsData=a_sinElecAngle_XA  IndexSearchMethod=Evenly spaced points  BeginIndexSearchUsingPreviousIndexResult=on  IndexDataTypeStr=uint8  RndMeth=Simplest
  r_sin3PhaA_M1 : Interpolation_n-D  NumberOfTableDimensions=1  Table=r_sin3PhaA_M1  ExtrapMethod=Clip  RemoveProtectionIndex=on  OutDataTypeStr=int16  InternalRulePriority=Speed  RndMeth=Simplest
      settings: InputPortMap=u0,u1
  r_sin3PhaB_M1 : Interpolation_n-D  NumberOfTableDimensions=1  Table=r_sin3PhaB_M1  ExtrapMethod=Clip  RemoveProtectionIndex=on  OutDataTypeStr=int16  InternalRulePriority=Speed  RndMeth=Simplest
      settings: InputPortMap=u0,u1
  r_sin3PhaC_M1 : Interpolation_n-D  NumberOfTableDimensions=1  Table=r_sin3PhaC_M1  ExtrapMethod=Clip  RemoveProtectionIndex=on  OutDataTypeStr=int16  InternalRulePriority=Speed  RndMeth=Simplest
      settings: InputPortMap=u0,u1
  r_phaA_Sin3 : Outport
  r_phaB_Sin3 : Outport  Port=2
  r_phaC_Sin3 : Outport  Port=3
  wires:
  a_sinElecAngle_XA/1 -> r_sin3PhaA_M1/1, r_sin3PhaC_M1/1, r_sin3PhaB_M1/1
  a_sinElecAngle_XA/2 -> r_sin3PhaC_M1/2, r_sin3PhaB_M1/2, r_sin3PhaA_M1/2
  r_sin3PhaA_M1/1 -> r_phaA_Sin3/1
  r_sin3PhaB_M1/1 -> r_phaB_Sin3/1
  r_sin3PhaC_M1/1 -> r_phaC_Sin3/1
  a_elecAngleAdv/1 -> a_sinElecAngle_XA/1

== system BLDC_controller_Lib_AccelerationBased/BLDC_controller/F03_Control_Method_Selection/signal_log1 ==
  r_phaB : Inport
  Terminator_1 : Terminator
  wires:
  r_phaB/1 -> Terminator_1/1  "r_phaB"

== system BLDC_controller_Lib_AccelerationBased/BLDC_controller/F03_Control_Method_Selection/signal_log2 ==
  r_phaC : Inport
  Terminator_1 : Terminator
  wires:
  r_phaC/1 -> Terminator_1/1  "r_phaC"

== system BLDC_controller_Lib_AccelerationBased/BLDC_controller/F03_Control_Method_Selection/signal_log6 ==
  r_phaA : Inport
  Terminator_1 : Terminator
  wires:
  r_phaA/1 -> Terminator_1/1  "r_phaA"

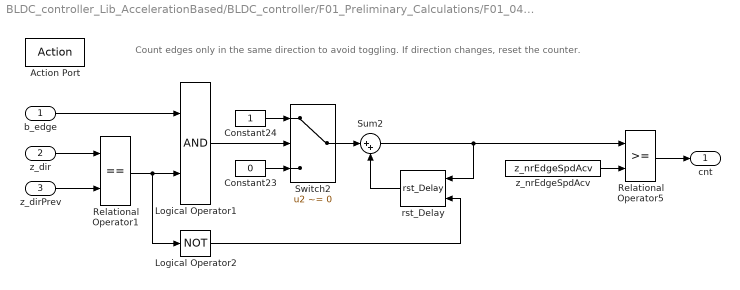
== system BLDC_controller_Lib_AccelerationBased/BLDC_controller/F01_Preliminary_Calculations/F01_04_Speed_Calculation/Edge_counter ==
  note: Count edges only in the same direction to avoid toggling. If direction changes, reset the counter.
  b_edge : Inport
  z_dir : Inport  Port=2
  z_dirPrev : Inport  Port=3
  Action Port : ActionPort
  Constant23 : Constant  Value=0  OutDataTypeStr=uint8
  Constant24 : Constant  OutDataTypeStr=uint8
  Logical Operator1 : Logic  AllPortsSameDT=off  OutDataTypeStr=boolean
  Logical Operator2 : Logic  Operator=NOT  AllPortsSameDT=off  OutDataTypeStr=boolean
  Relational Operator1 : RelationalOperator  Operator===  OutDataTypeStr=boolean  RndMeth=Simplest
  Relational Operator5 : RelationalOperator  OutDataTypeStr=boolean  RndMeth=Simplest
  Sum2 : Sum  Inputs=|++  InputSameDT=on  OutDataTypeStr=Inherit: Same as first input
  Switch2 : Switch  Criteria=u2 ~= 0  OutDataTypeStr=Inherit: Inherit via back propagation  RndMeth=Simplest
  rst_Delay : BLDC_controller_Lib/rst_Delay
  z_nrEdgeSpdAcv : Constant  Value=z_nrEdgeSpdAcv  OutDataTypeStr=Inherit: Inherit via back propagation
  cnt : Outport  OutputWhenDisabled=reset  InitialOutput=0
  wires:
  Relational Operator5/1 -> cnt/1
  z_nrEdgeSpdAcv/1 -> Relational Operator5/2
  Sum2/1 -> rst_Delay/1, Relational Operator5/1
  Switch2/1 -> Sum2/1
  Constant23/1 -> Switch2/3
  Constant24/1 -> Switch2/1
  rst_Delay/1 -> Sum2/2
  Relational Operator1/1 -> Logical Operator2/1, Logical Operator1/2
  z_dir/1 -> Relational Operator1/1
  z_dirPrev/1 -> Relational Operator1/2
  Logical Operator2/1 -> rst_Delay/2
  b_edge/1 -> Logical Operator1/1
  Logical Operator1/1 -> Switch2/2

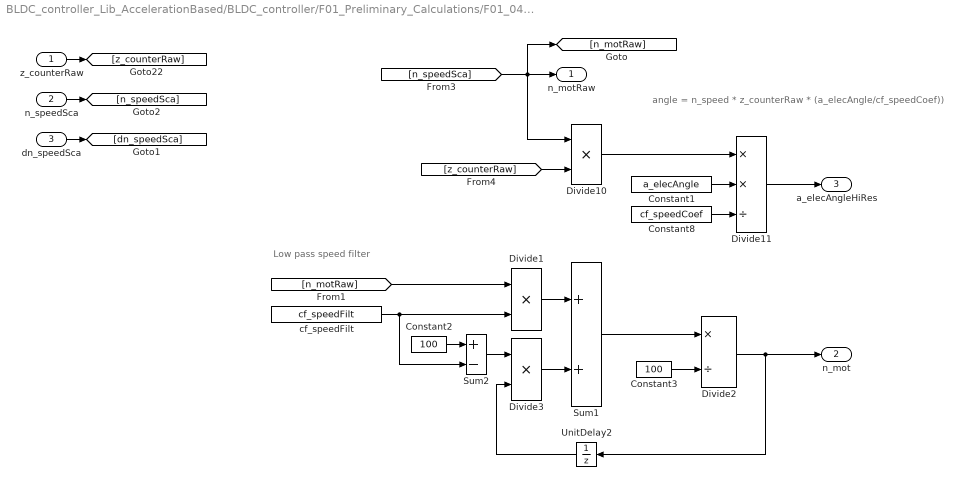
== system BLDC_controller_Lib_AccelerationBased/BLDC_controller/F01_Preliminary_Calculations/F01_04_Speed_Calculation/Final_Motor_Speed_Calculation ==
  note: Low pass speed filter
  note: angle = n_speed * z_counterRaw * (a_elecAngle/cf_speedCoef))
  z_counterRaw : Inport
  n_speedSca : Inport  Port=2
  dn_speedSca : Inport  Port=3
  Constant1 : Constant  Value=a_elecAngle  OutDataTypeStr=Inherit: Inherit via back propagation
  Constant2 : Constant  Value=100  OutDataTypeStr=Inherit: Inherit via back propagation
  Constant3 : Constant  Value=100  OutDataTypeStr=Inherit: Inherit via back propagation
  Constant8 : Constant  Value=cf_speedCoef  OutDataTypeStr=Inherit: Inherit via back propagation
  Divide1 : Product  Inputs=**  RndMeth=Simplest  OutDataTypeStr=Inherit: Same as first input
  Divide10 : Product  Inputs=**  RndMeth=Simplest  OutDataTypeStr=Inherit: Same as first input
  Divide11 : Product  Inputs=**/  RndMeth=Simplest  SaturateOnIntegerOverflow=on  OutDataTypeStr=Inherit: Same as first input
  Divide2 : Product  Inputs=*/  RndMeth=Simplest  OutDataTypeStr=Inherit: Same as first input
  Divide3 : Product  Inputs=**  RndMeth=Simplest  OutDataTypeStr=Inherit: Same as first input
  Sum1 : Sum  RndMeth=Simplest  InputSameDT=on  OutDataTypeStr=Inherit: Same as first input
  Sum2 : Sum  Inputs=+-  RndMeth=Simplest  InputSameDT=on  OutDataTypeStr=Inherit: Same as first input
  UnitDelay2 : UnitDelay  SampleTime=-1
  cf_speedFilt : Constant  Value=cf_speedFilt  OutDataTypeStr=int32
  n_motRaw : Outport
  n_mot : Outport  Port=2
  a_elecAngleHiRes : Outport  Port=3
  wires:
  [z_counterRaw] -> Divide10/2
  Divide11/1 -> a_elecAngleHiRes/1
  Constant1/1 -> Divide11/2
  Constant8/1 -> Divide11/3
  Divide10/1 -> Divide11/1
  [n_speedSca] -> [n_motRaw], Divide10/1, n_motRaw/1
  n_speedSca/1 -> [n_speedSca]
  dn_speedSca/1 -> [dn_speedSca]
  z_counterRaw/1 -> [z_counterRaw]
  Constant3/1 -> Divide2/2
  Sum1/1 -> Divide2/1
  Divide2/1 -> UnitDelay2/1, n_mot/1
  Divide1/1 -> Sum1/1
  UnitDelay2/1 -> Divide3/2
  Divide3/1 -> Sum1/2
  Constant2/1 -> Sum2/1
  Sum2/1 -> Divide3/1
  cf_speedFilt/1 -> Sum2/2, Divide1/2
  [n_motRaw] -> Divide1/1

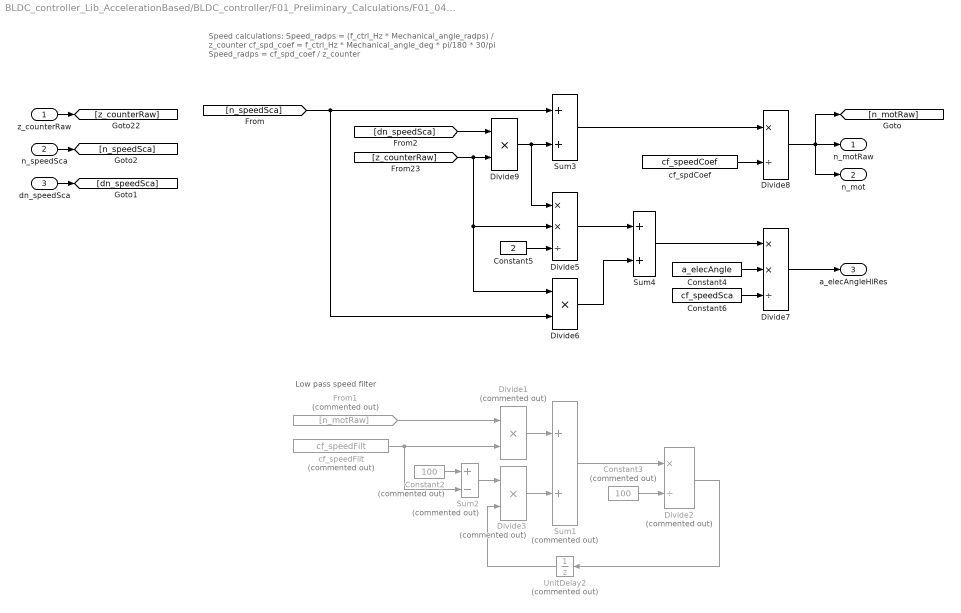
== system BLDC_controller_Lib_AccelerationBased/BLDC_controller/F01_Preliminary_Calculations/F01_04_Speed_Calculation/Final_Motor_Speed_Calculation1 ==
  note: Low pass speed filter
  note: Speed calculations:
      | Speed_radps = (f_ctrl_Hz * Mechanical_angle_radps) / z_counter
      | cf_spd_coef = f_ctrl_Hz * Mechanical_angle_deg * pi/180 * 30/pi
      | Speed_radps = cf_spd_coef / z_counter
  z_counterRaw : Inport
  n_speedSca : Inport  Port=2
  dn_speedSca : Inport  Port=3
  Constant2 : Constant  Commented=on  Value=100  OutDataTypeStr=Inherit: Inherit via back propagation
  Constant3 : Constant  Commented=on  Value=100  OutDataTypeStr=Inherit: Inherit via back propagation
  Constant4 : Constant  Value=a_elecAngle  OutDataTypeStr=Inherit: Inherit via back propagation
  Constant5 : Constant  Value=2  OutDataTypeStr=Inherit: Inherit via back propagation
  Constant6 : Constant  Value=cf_speedSca  OutDataTypeStr=Inherit: Inherit via back propagation
  Divide1 : Product  Commented=on  Inputs=**  RndMeth=Simplest  OutDataTypeStr=Inherit: Same as first input
  Divide2 : Product  Commented=on  Inputs=*/  RndMeth=Simplest  OutDataTypeStr=Inherit: Same as first input
  Divide3 : Product  Commented=on  Inputs=**  RndMeth=Simplest  OutDataTypeStr=Inherit: Same as first input
  Divide5 : Product  Inputs=**/  RndMeth=Simplest  OutDataTypeStr=Inherit: Same as first input
  Divide6 : Product  Inputs=**  RndMeth=Simplest  OutDataTypeStr=Inherit: Same as first input
  Divide7 : Product  Inputs=**/  RndMeth=Simplest  SaturateOnIntegerOverflow=on  OutDataTypeStr=Inherit: Same as first input
  Divide8 : Product  Inputs=*/  RndMeth=Simplest  OutDataTypeStr=Inherit: Same as first input
  Divide9 : Product  Inputs=**  RndMeth=Simplest  OutDataTypeStr=Inherit: Same as first input
  From1 : From  Commented=on  GotoTag=n_motRaw
  Sum1 : Sum  Commented=on  RndMeth=Simplest  InputSameDT=on  OutDataTypeStr=Inherit: Same as first input
  Sum2 : Sum  Commented=on  Inputs=+-  RndMeth=Simplest  InputSameDT=on  OutDataTypeStr=Inherit: Same as first input
  Sum3 : Sum  RndMeth=Simplest  InputSameDT=on  OutDataTypeStr=Inherit: Same as first input
  Sum4 : Sum  RndMeth=Simplest  InputSameDT=on  OutDataTypeStr=Inherit: Same as first input
  UnitDelay2 : UnitDelay  Commented=on  SampleTime=-1
  cf_spdCoef : Constant  Value=cf_speedCoef  OutDataTypeStr=int32
  cf_speedFilt : Constant  Commented=on  Value=cf_speedFilt  OutDataTypeStr=int32
  n_motRaw : Outport
  n_mot : Outport  Port=2
  a_elecAngleHiRes : Outport  Port=3
  wires:
  From1/1 -> Divide1/1
  cf_speedFilt/1 -> Divide1/2, Sum2/2
  Sum2/1 -> Divide3/1
  Constant2/1 -> Sum2/1
  Divide3/1 -> Sum1/2
  UnitDelay2/1 -> Divide3/2
  Divide1/1 -> Sum1/1
  Divide2/1 -> UnitDelay2/1
  Sum1/1 -> Divide2/1
  Constant3/1 -> Divide2/2
  Sum3/1 -> Divide8/1
  [z_counterRaw] -> Divide6/1, Divide5/2, Divide9/2
  Divide6/1 -> Sum4/2
  Constant4/1 -> Divide7/2
  [dn_speedSca] -> Divide9/1
  [n_speedSca] -> Divide6/2, Sum3/1
  Sum4/1 -> Divide7/1
  cf_spdCoef/1 -> Divide8/2
  Divide5/1 -> Sum4/1
  Constant6/1 -> Divide7/3
  Constant5/1 -> Divide5/3
  z_counterRaw/1 -> [z_counterRaw]
  dn_speedSca/1 -> [dn_speedSca]
  n_speedSca/1 -> [n_speedSca]
  Divide8/1 -> [n_motRaw], n_motRaw/1, n_mot/1
  Divide9/1 -> Divide5/1, Sum3/2
  Divide7/1 -> a_elecAngleHiRes/1

== system BLDC_controller_Lib_AccelerationBased/BLDC_controller/F01_Preliminary_Calculations/F01_04_Speed_Calculation/Speed_and_Acceleration_Calculation ==
  note: Speed calculations:
      | Speed_radps = (f_ctrl_Hz * Mechanical_angle_radps) / z_counter
      | cf_spd_coef = f_ctrl_Hz * Mechanical_angle_deg * pi/180 * 30/pi
      | Speed_radps = cf_spd_coef / z_counter
  note: Counter error calculation. In case the calculation is not enabled output 0.
  b_cntEna : Inport
  z_dir : Inport  Port=2
  z_counter : Inport  Port=3
  Trigger : TriggerPort  VariantControl=Variant  ZeroCross=off  PortDimensions=1
  Constant1 : Constant  Value=0  OutDataTypeStr=Inherit: Inherit via back propagation
  Constant3 : Constant  Value=cf_speedCoef  OutDataTypeStr=Inherit: Inherit via back propagation
  Divide2 : Product  Inputs=**/  RndMeth=Simplest  OutDataTypeStr=Inherit: Same as first input
  Switch : Switch  Criteria=u2 ~= 0  OutDataTypeStr=Inherit: Inherit via back propagation  RndMeth=Simplest
  n_speedSca : Outport
  wires:
  Switch/1 -> n_speedSca/1
  [z_dir] -> Divide2/2
  z_dir/1 -> [z_dir]
  z_counter/1 -> [z_counter]
  b_cntEna/1 -> [b_cntEna]
  Divide2/1 -> Switch/1
  Constant3/1 -> Divide2/1
  [z_counter] -> Divide2/3
  Constant1/1 -> Switch/3
  [b_cntEna] -> Switch/2

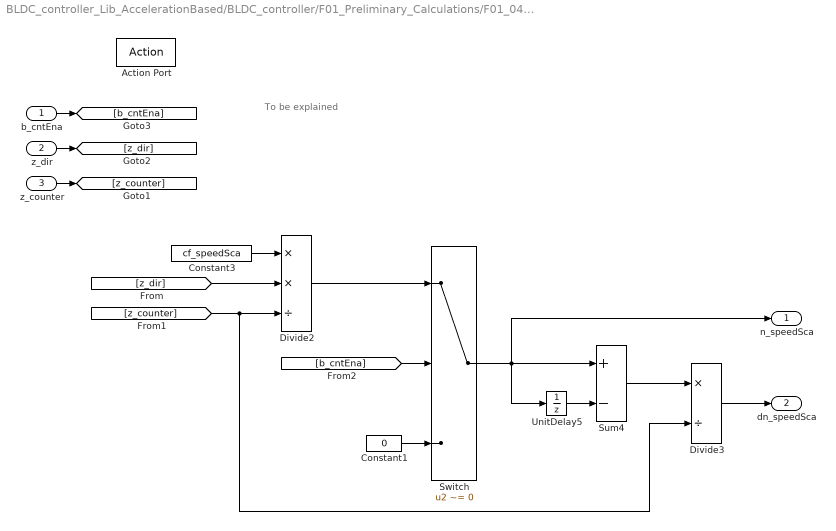
== system BLDC_controller_Lib_AccelerationBased/BLDC_controller/F01_Preliminary_Calculations/F01_04_Speed_Calculation/Speed_and_Acceleration_Calculation1 ==
  note: To be explained
  b_cntEna : Inport
  z_dir : Inport  Port=2
  z_counter : Inport  Port=3
  Action Port : ActionPort
  Constant1 : Constant  Value=0  OutDataTypeStr=Inherit: Inherit via back propagation
  Constant3 : Constant  Value=cf_speedSca  OutDataTypeStr=Inherit: Inherit via back propagation
  Divide2 : Product  Inputs=**/  RndMeth=Simplest  OutDataTypeStr=Inherit: Same as first input
  Divide3 : Product  Inputs=*/  RndMeth=Simplest  OutDataTypeStr=Inherit: Same as first input
  Sum4 : Sum  Inputs=+-  RndMeth=Simplest  InputSameDT=on  OutDataTypeStr=Inherit: Same as first input
  Switch : Switch  Criteria=u2 ~= 0  OutDataTypeStr=Inherit: Inherit via back propagation  RndMeth=Simplest
  UnitDelay5 : UnitDelay  SampleTime=-1
  n_speedSca : Outport
  dn_speedSca : Outport  Port=2
  wires:
  Divide3/1 -> dn_speedSca/1
  [b_cntEna] -> Switch/2
  Constant1/1 -> Switch/3
  [z_counter] -> Divide3/2, Divide2/3
  Constant3/1 -> Divide2/1
  Switch/1 -> Sum4/1, UnitDelay5/1, n_speedSca/1
  Sum4/1 -> Divide3/1
  UnitDelay5/1 -> Sum4/2
  Divide2/1 -> Switch/1
  b_cntEna/1 -> [b_cntEna]
  z_counter/1 -> [z_counter]
  z_dir/1 -> [z_dir]
  [z_dir] -> Divide2/2
